simulink model "quad_1_ref_NN"  (R2018b)
settings: Solver=VariableStepAuto  StartTime=0.0  StopTime=20  RelTol=1e-3
undefined symbols (not defined in the file or in its folder): options
libraries: neural x348, simulink x3
(part 5 of 13)

== system quad_1_ref_NN/nn_1/Layer 3/Delays 1 ==
  "p{3}" : Inport  PortDimensions=30
      mask Display: e = 0.06;c1 = [120 230 180]/255;c2 = ([120 230 180]+0)/(256+128);c3 = ([120 230 180]+128)/(256+128);patch([0 1 1 0],[0 0 1 1],c1);patch([0 1 1 1-e 1-e 0+e],[0 0 1 1-e 0+e 0+e],c2);patch([0 0 1 1-e 0+e 0+e],[0 1 1 1-e 1-e 0+e],c3);plot([0 1 1 0 0],[0 0 1 1 0]);
  mux : Mux  Inputs=1
      mask Display: e = 0.06;c1 = [120 150 230]/255;c2 = ([120 150 230]+0)/383;c3 = ([120 150 230]+128)/383;patch([0 1 1 0],[0 0 1 1],c1);patch([0 1 1 1-e 1-e 0+e],[0 0 1 1-e 0+e 0+e],c2);patch([0 0 1 1-e 0+e 0+e],[0 1 1 1-e 1-e 0+e],c3);plot([0 1 1 0 0],[0 0 1 1 0]);disp('Mux')
  "pd{3,2}" : Outport
      mask Display: e = 0.06;c1 = [120 230 180]/255;c2 = ([120 230 180]+0)/(256+128);c3 = ([120 230 180]+128)/(256+128);patch([0 1 1 0],[0 0 1 1],c1);patch([0 1 1 1-e 1-e 0+e],[0 0 1 1-e 0+e 0+e],c2);patch([0 0 1 1-e 0+e 0+e],[0 1 1 1-e 1-e 0+e],c3);plot([0 1 1 0 0],[0 0 1 1 0]);
  wires:
  "p{3}"/1 -> mux/1
  mux/1 -> "pd{3,2}"/1

== system quad_1_ref_NN/nn_1/Layer 3/LW{3,2} ==
  "ad{3,2}" : Inport  PortDimensions=30
      mask Display: e = 0.06;c1 = [120 230 180]/255;c2 = ([120 230 180]+0)/(256+128);c3 = ([120 230 180]+128)/(256+128);patch([0 1 1 0],[0 0 1 1],c1);patch([0 1 1 1-e 1-e 0+e],[0 0 1 1-e 0+e 0+e],c2);patch([0 0 1 1-e 0+e 0+e],[0 1 1 1-e 1-e 0+e],c3);plot([0 1 1 0 0],[0 0 1 1 0]);
  "IW{3,2}(1,:)'" : Constant  Value=[0.276945469071661454218968856366700492799282073974609375;-0.30202511226643291575300054319086484611034393310546875;-0.20444458747253602126647820114158093929290771484375;-0.293398521295770098316069152133422903716564178466796875;-0.311767883755503738552050663201953284442424774169921875;0.2018687666357379117965109571741777472198009490966796875;-0.1423334383288296922653870524300145916640758514404296875;0.042721362346013591615445648130844347178936004638671875;-0.2329868918425182788833893710034317336976528167724609375;0.3249510619125837163068126756115816533565521240234375;-0.236296700940786752465072595441597513854503631591796875;0.0895607189297012162843003579837386496365070343017578125;0.12291057624967384465097808288192027248442173004150390625;-0.23707638583951962107931876744260080158710479736328125;-0.0601267258706521812161582829503458924591541290283203125;0.0826306713186458485775887083946145139634609222412109375;0.180972528352075279212129998995806090533733367919921875;-0.1529426971898099341107268855921574868261814117431640625;-0.2028170626333564430243683318622061051428318023681640625;0.1491957272053341110318314122196170501410961151123046875;0.170336272776724972910500355283147655427455902099609375;-0.28514001098319774474276755427126772701740264892578125;-0.1635604930433562642644318430029670707881450653076171875;0.360323245380352485955910424308967776596546173095703125;-0.349567524080722058510417582510854117572307586669921875;0.230681480735392574477060634308145381510257720947265625;0.2623154158955223191895811396534554660320281982421875;0.039798895545825989372712427893929998390376567840576171875;0.1587870984716829581007146998672396875917911529541015625;-0.26822414961531659827187468181364238262176513671875]
      mask Display: e = 0.06;c1 = [120 150 230]/255;c2 = ([120 150 230]+0)/383;c3 = ([120 150 230]+128)/383;patch([0 1 1 0],[0 0 1 1],c1);patch([0 1 1 1-e 1-e 0+e],[0 0 1 1-e 0+e 0+e],c2);patch([0 0 1 1-e 0+e 0+e],[0 1 1 1-e 1-e 0+e],c3);plot([0 1 1 0 0],[0 0 1 1 0]);disp('weights');
  "IW{3,2}(2,:)'" : Constant  Value=[-0.03253994981968925948034865314184571616351604461669921875;0.0550317097961975643105603239746415056288242340087890625;0.00642099379508191507592851365870956215076148509979248046875;0.03913085661204451781713942182250320911407470703125;-0.00475663585868581727245096857359385467134416103363037109375;-0.01086399947620869492481698870278705726377665996551513671875;0.0311382195567674602276753148544230498373508453369140625;-0.00372679100208476825339953819593574735336005687713623046875;-0.002270132986024297160054796762551632127724587917327880859375;0.020055220330963123565037875550842727534472942352294921875;0.0131234617942851128358228152137598954141139984130859375;0.0034257306991433904112820396647975940140895545482635498046875;-0.002660691719241682455521225136862994986586272716522216796875;0.0037828286499629027415936288747388971387408673763275146484375;-0.020157961923446821028704789569019339978694915771484375;-0.05222008698724234232457774851354770362377166748046875;-0.0196956397109985283100375141884796903468668460845947265625;0.021014223419305817774915823292758432216942310333251953125;-0.028243561683475686130417869890152360312640666961669921875;-0.0217372382094138498487279065329857985489070415496826171875;-0.0135213933507876242490208795743455993942916393280029296875;-0.00476408825410913443210159101681711035780608654022216796875;-0.00653767842271109345109181276711751706898212432861328125;-0.000516617713027289586491530570810937206260859966278076171875;0.024000774270628875972644067360306507907807826995849609375;0.01625825744361460156728327319797244854271411895751953125;-0.0030105080437037141059819500554795013158582150936126708984375;-0.0178769935667331854312056549360931967385113239288330078125;0.0523806529586079150373478796609560959041118621826171875;-0.0290655000588837496289240647229235037229955196380615234375]
      mask Display: e = 0.06;c1 = [120 150 230]/255;c2 = ([120 150 230]+0)/383;c3 = ([120 150 230]+128)/383;patch([0 1 1 0],[0 0 1 1],c1);patch([0 1 1 1-e 1-e 0+e],[0 0 1 1-e 0+e 0+e],c2);patch([0 0 1 1-e 0+e 0+e],[0 1 1 1-e 1-e 0+e],c3);plot([0 1 1 0 0],[0 0 1 1 0]);disp('weights');
  "IW{3,2}(3,:)'" : Constant  Value=[-0.009031921548045683534322591867748997174203395843505859375;0.05112964354185862980717303116762195713818073272705078125;0.022652209907742172634304012035499908961355686187744140625;0.04418223617098011868353779618701082654297351837158203125;-0.03234466873359742589144616431440226733684539794921875;0.0062948422769956470512742185974275344051420688629150390625;0.0075733059480824101161733352682858821935951709747314453125;-0.0031465398829118623909295582308232042123563587665557861328125;0.0257908390726858359476292292811194784007966518402099609375;0.01442129708941418224366071143549561384133994579315185546875;-0.003383104425635254097759485603091889061033725738525390625;0.01580392529714715055266793797272839583456516265869140625;-0.0310251890936021727795957048101627151481807231903076171875;-0.01179788359657658360080123571833610185422003269195556640625;-0.010215859514722404333131322573535726405680179595947265625;-0.05484074893927239069402190807522856630384922027587890625;-0.013821153985895277827022908923026989214122295379638671875;0.025982866454749765916520942710121744312345981597900390625;-0.021905026659969996372101519455100060440599918365478515625;-0.0526800415654134768228544771773158572614192962646484375;0.01189509994522582568554636139879221445880830287933349609375;0.01084111337574418000573306386513650068081915378570556640625;-0.00337372300491556829926675931119461893104016780853271484375;0.00449380387199421228727747035236461670137941837310791015625;0.0106078987897606606682909813343940186314284801483154296875;-0.00067881771438273175167665840490371920168399810791015625;-0.00932376731050502290110149061774791334755718708038330078125;-0.0245059899770730983681321646372452960349619388580322265625;0.019977292170611275767821979343352722935378551483154296875;-0.04273760279662632000086119887782842852175235748291015625]
      mask Display: e = 0.06;c1 = [120 150 230]/255;c2 = ([120 150 230]+0)/383;c3 = ([120 150 230]+128)/383;patch([0 1 1 0],[0 0 1 1],c1);patch([0 1 1 1-e 1-e 0+e],[0 0 1 1-e 0+e 0+e],c2);patch([0 0 1 1-e 0+e 0+e],[0 1 1 1-e 1-e 0+e],c3);plot([0 1 1 0 0],[0 0 1 1 0]);disp('weights');
  Mux : Mux  Inputs=3
      mask Display: e = 0.06;c1 = [120 150 230]/255;c2 = ([120 150 230]+0)/383;c3 = ([120 150 230]+128)/383;patch([0 1 1 0],[0 0 1 1],c1);patch([0 1 1 1-e 1-e 0+e],[0 0 1 1-e 0+e 0+e],c2);patch([0 0 1 1-e 0+e 0+e],[0 1 1 1-e 1-e 0+e],c3);plot([0 1 1 0 0],[0 0 1 1 0]);disp('Mux');
  dotprod1 : neural/Weight Functions/dotprod
  dotprod2 : neural/Weight Functions/dotprod
  dotprod3 : neural/Weight Functions/dotprod
  "lz{3,2}" : Outport
      mask Display: e = 0.06;c1 = [120 230 180]/255;c2 = ([120 230 180]+0)/(256+128);c3 = ([120 230 180]+128)/(256+128);patch([0 1 1 0],[0 0 1 1],c1);patch([0 1 1 1-e 1-e 0+e],[0 0 1 1-e 0+e 0+e],c2);patch([0 0 1 1-e 0+e 0+e],[0 1 1 1-e 1-e 0+e],c3);plot([0 1 1 0 0],[0 0 1 1 0]);
  wires:
  "IW{3,2}(1,:)'"/1 -> dotprod1/1
  "ad{3,2}"/1 -> dotprod1/2, dotprod2/2, dotprod3/2
  dotprod1/1 -> Mux/1
  "IW{3,2}(2,:)'"/1 -> dotprod2/1
  dotprod2/1 -> Mux/2
  "IW{3,2}(3,:)'"/1 -> dotprod3/1
  dotprod3/1 -> Mux/3
  Mux/1 -> "lz{3,2}"/1

== system quad_1_ref_NN/nn_1_const/Layer 1/Delays 1 ==
  "p{1}" : Inport  PortDimensions=12
      mask Display: e = 0.06;c1 = [120 230 180]/255;c2 = ([120 230 180]+0)/(256+128);c3 = ([120 230 180]+128)/(256+128);patch([0 1 1 0],[0 0 1 1],c1);patch([0 1 1 1-e 1-e 0+e],[0 0 1 1-e 0+e 0+e],c2);patch([0 0 1 1-e 0+e 0+e],[0 1 1 1-e 1-e 0+e],c3);plot([0 1 1 0 0],[0 0 1 1 0]);
  mux : Mux  Inputs=1
      mask Display: e = 0.06;c1 = [120 150 230]/255;c2 = ([120 150 230]+0)/383;c3 = ([120 150 230]+128)/383;patch([0 1 1 0],[0 0 1 1],c1);patch([0 1 1 1-e 1-e 0+e],[0 0 1 1-e 0+e 0+e],c2);patch([0 0 1 1-e 0+e 0+e],[0 1 1 1-e 1-e 0+e],c3);plot([0 1 1 0 0],[0 0 1 1 0]);disp('Mux')
  "pd{1,1}" : Outport
      mask Display: e = 0.06;c1 = [120 230 180]/255;c2 = ([120 230 180]+0)/(256+128);c3 = ([120 230 180]+128)/(256+128);patch([0 1 1 0],[0 0 1 1],c1);patch([0 1 1 1-e 1-e 0+e],[0 0 1 1-e 0+e 0+e],c2);patch([0 0 1 1-e 0+e 0+e],[0 1 1 1-e 1-e 0+e],c3);plot([0 1 1 0 0],[0 0 1 1 0]);
  wires:
  "p{1}"/1 -> mux/1
  mux/1 -> "pd{1,1}"/1

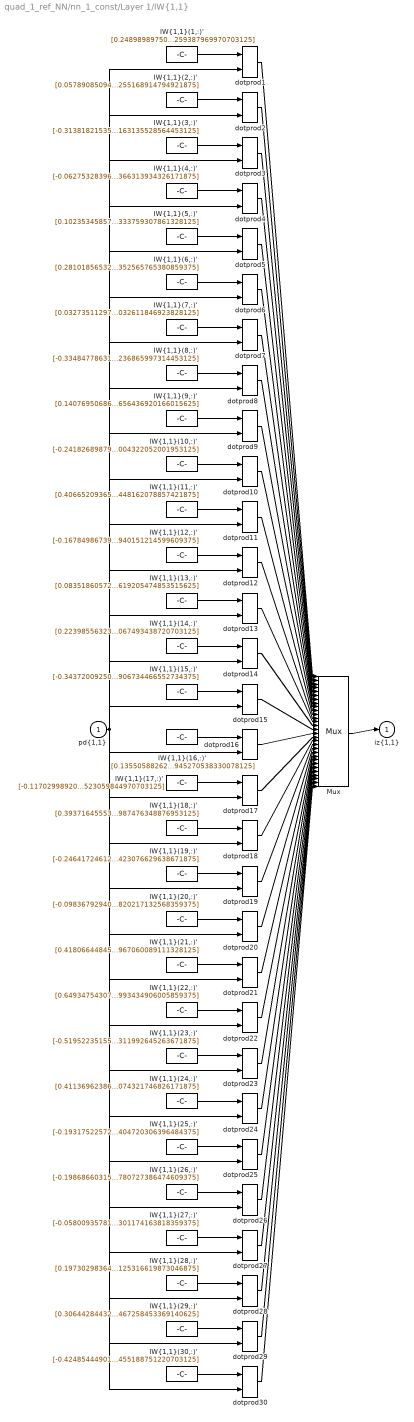
== system quad_1_ref_NN/nn_1_const/Layer 1/IW{1,1} ==
  "pd{1,1}" : Inport  PortDimensions=12
      mask Display: e = 0.06;c1 = [120 230 180]/255;c2 = ([120 230 180]+0)/(256+128);c3 = ([120 230 180]+128)/(256+128);patch([0 1 1 0],[0 0 1 1],c1);patch([0 1 1 1-e 1-e 0+e],[0 0 1 1-e 0+e 0+e],c2);patch([0 0 1 1-e 0+e 0+e],[0 1 1 1-e 1-e 0+e],c3);plot([0 1 1 0 0],[0 0 1 1 0]);
  "IW{1,1}(1,:)'" : Constant  Value=[0.2489898975063435937471467696013860404491424560546875;-0.112298286921174328423234101137495599687099456787109375;-0.041923837097128206774510061904948088340461254119873046875;-0.046673404176335420157073485825094394385814666748046875;0.432665213666946379955646762027754448354244232177734375;-0.0097132578185999095266023317662984482012689113616943359375;0.32656184582790304116173274451284669339656829833984375;0.11158683144684687638115150321027613244950771331787109375;-0.00174609248808417038927032205464229264180175960063934326171875;0.424027280725470578914837460615672171115875244140625;0.458406862610547083392020795145072042942047119140625;-0.0370983845065871176149840948710334487259387969970703125]
      mask Display: e = 0.06;c1 = [120 150 230]/255;c2 = ([120 150 230]+0)/383;c3 = ([120 150 230]+128)/383;patch([0 1 1 0],[0 0 1 1],c1);patch([0 1 1 1-e 1-e 0+e],[0 0 1 1-e 0+e 0+e],c2);patch([0 0 1 1-e 0+e 0+e],[0 1 1 1-e 1-e 0+e],c3);plot([0 1 1 0 0],[0 0 1 1 0]);disp('Weights');
  "IW{1,1}(10,:)'" : Constant  Value=[-0.241826898792885547351261266157962381839752197265625;0.3919254723671212747859726732713170349597930908203125;-0.0213357064703371020197852914179748040623962879180908203125;-0.09792977901171183441331180574707104824483394622802734375;0.047839481153725486872740901844736072234809398651123046875;0.116526714482541871031884284093393944203853607177734375;-0.0918185950644110626672755870458786375820636749267578125;-0.197897683283946912435879994518472813069820404052734375;-0.0712123900064262349562937970404163934290409088134765625;-0.34083989126823810433819517129450105130672454833984375;-0.56405002922402591725159481939044781029224395751953125;0.031834197805936444158891873712491360493004322052001953125]
      mask Display: e = 0.06;c1 = [120 150 230]/255;c2 = ([120 150 230]+0)/383;c3 = ([120 150 230]+128)/383;patch([0 1 1 0],[0 0 1 1],c1);patch([0 1 1 1-e 1-e 0+e],[0 0 1 1-e 0+e 0+e],c2);patch([0 0 1 1-e 0+e 0+e],[0 1 1 1-e 1-e 0+e],c3);plot([0 1 1 0 0],[0 0 1 1 0]);disp('Weights');
  "IW{1,1}(11,:)'" : Constant  Value=[0.406652093651284685105196103904745541512966156005859375;-0.276759606675215596993666622438468039035797119140625;-0.1913370529300668920757999558190931566059589385986328125;0.311012617222419240903263926156796514987945556640625;-0.18175282140661253027502652912517078220844268798828125;-0.05621199948579279348503945357151678763329982757568359375;0.207761145657090418037427070885314606130123138427734375;0.29617604491022142543243944601272232830524444580078125;-0.2494736920950384462258853091043420135974884033203125;-0.398387101331069859444511394030996598303318023681640625;0.37593373815508146496000563274719752371311187744140625;0.0935813620128422563038128600965137593448162078857421875]
      mask Display: e = 0.06;c1 = [120 150 230]/255;c2 = ([120 150 230]+0)/383;c3 = ([120 150 230]+128)/383;patch([0 1 1 0],[0 0 1 1],c1);patch([0 1 1 1-e 1-e 0+e],[0 0 1 1-e 0+e 0+e],c2);patch([0 0 1 1-e 0+e 0+e],[0 1 1 1-e 1-e 0+e],c3);plot([0 1 1 0 0],[0 0 1 1 0]);disp('Weights');
  "IW{1,1}(12,:)'" : Constant  Value=[-0.1678498673909872007659060955120366998016834259033203125;0.30057791076311601852211197183351032435894012451171875;-0.2068623881193169811165688543042051605880260467529296875;0.03127024359038514667030739246911252848803997039794921875;-0.275997240372790997309238036905298940837383270263671875;0.366594694572909662877435721384244970977306365966796875;0.4295578731804960970208639992051757872104644775390625;0.327463701071572355072447635393473319709300994873046875;-0.193276403110250794004087993016582913696765899658203125;-0.345485768180975372221297448049881495535373687744140625;-0.1335022226039513648654377675484283827245235443115234375;0.1217009352881620320996347572872764430940151214599609375]
      mask Display: e = 0.06;c1 = [120 150 230]/255;c2 = ([120 150 230]+0)/383;c3 = ([120 150 230]+128)/383;patch([0 1 1 0],[0 0 1 1],c1);patch([0 1 1 1-e 1-e 0+e],[0 0 1 1-e 0+e 0+e],c2);patch([0 0 1 1-e 0+e 0+e],[0 1 1 1-e 1-e 0+e],c3);plot([0 1 1 0 0],[0 0 1 1 0]);disp('Weights');
  "IW{1,1}(13,:)'" : Constant  Value=[0.08351860572411019811855936723077320493757724761962890625;-0.413325214603568025228952365068835206329822540283203125;-0.302060946120565165795568418616312555968761444091796875;-0.116192348966924707820425055615487508475780487060546875;-0.149872004616036225144171112333424389362335205078125;0.3732993546496150560898286130395717918872833251953125;-0.44533869376238433002157535156584344804286956787109375;0.0395748086544917831997025814416701905429363250732421875;0.1197405812416630632721847860011621378362178802490234375;-0.41575965708720274971454955448280088603496551513671875;-0.2246661150830329967131859802975668571889400482177734375;-0.0216388332703475738671983208405436016619205474853515625]
      mask Display: e = 0.06;c1 = [120 150 230]/255;c2 = ([120 150 230]+0)/383;c3 = ([120 150 230]+128)/383;patch([0 1 1 0],[0 0 1 1],c1);patch([0 1 1 1-e 1-e 0+e],[0 0 1 1-e 0+e 0+e],c2);patch([0 0 1 1-e 0+e 0+e],[0 1 1 1-e 1-e 0+e],c3);plot([0 1 1 0 0],[0 0 1 1 0]);disp('Weights');
  "IW{1,1}(14,:)'" : Constant  Value=[0.223985563232536766253844007223960943520069122314453125;-0.04945192503423155583330839135669521056115627288818359375;-0.1962965394305775934657987136233714409172534942626953125;0.0295316519582797358534076437308613094501197338104248046875;0.07949822490435536070929600782619672827422618865966796875;-0.51816763343045213474624688387848436832427978515625;0.10949461368816186535024570503082941286265850067138671875;-0.01143505829141123163184001754189011990092694759368896484375;0.582963912201748701846781841595657169818878173828125;0.0268494871259278948538717912697393330745398998260498046875;0.0069103283755132215160355002581127337180078029632568359375;-0.4759050293050759439239527637255378067493438720703125]
      mask Display: e = 0.06;c1 = [120 150 230]/255;c2 = ([120 150 230]+0)/383;c3 = ([120 150 230]+128)/383;patch([0 1 1 0],[0 0 1 1],c1);patch([0 1 1 1-e 1-e 0+e],[0 0 1 1-e 0+e 0+e],c2);patch([0 0 1 1-e 0+e 0+e],[0 1 1 1-e 1-e 0+e],c3);plot([0 1 1 0 0],[0 0 1 1 0]);disp('Weights');
  "IW{1,1}(15,:)'" : Constant  Value=[-0.34372009250453372519729100531549192965030670166015625;-0.3295648638163488630681285940227098762989044189453125;-0.26076996190842560707778829964809119701385498046875;-0.0354217042376119561897240828329813666641712188720703125;-0.32720899914815737563600350767956115305423736572265625;-0.2344401070546141274686391398063278757035732269287109375;-0.340184475584872914044609615302761085331439971923828125;-0.27627829555073779577156756204203702509403228759765625;0.1048058417402470687829207918184692971408367156982421875;-0.15736575485780124328272222555824555456638336181640625;0.334995769922207198288077734105172567069530487060546875;0.1470607822368401595980458296253345906734466552734375]
      mask Display: e = 0.06;c1 = [120 150 230]/255;c2 = ([120 150 230]+0)/383;c3 = ([120 150 230]+128)/383;patch([0 1 1 0],[0 0 1 1],c1);patch([0 1 1 1-e 1-e 0+e],[0 0 1 1-e 0+e 0+e],c2);patch([0 0 1 1-e 0+e 0+e],[0 1 1 1-e 1-e 0+e],c3);plot([0 1 1 0 0],[0 0 1 1 0]);disp('Weights');
  "IW{1,1}(16,:)'" : Constant  Value=[0.1355058826287278972433369972350192256271839141845703125;-0.327508281343989182676779137182165868580341339111328125;-0.162426252210169097534020465900539420545101165771484375;-0.379662675760057855001150528551079332828521728515625;-0.02615657306319595087895635288077755831182003021240234375;0.2034431436294713291257352238972089253365993499755859375;0.0037668162158365713597374391241601188085041940212249755859375;-0.386785824856337001609318804185022599995136260986328125;-0.08908442379376861619544314407903584651648998260498046875;0.419719320235534099072793878804077394306659698486328125;-0.394700658331529175004703802187577821314334869384765625;0.06888911276263716410017678981603239662945270538330078125]
      mask Display: e = 0.06;c1 = [120 150 230]/255;c2 = ([120 150 230]+0)/383;c3 = ([120 150 230]+128)/383;patch([0 1 1 0],[0 0 1 1],c1);patch([0 1 1 1-e 1-e 0+e],[0 0 1 1-e 0+e 0+e],c2);patch([0 0 1 1-e 0+e 0+e],[0 1 1 1-e 1-e 0+e],c3);plot([0 1 1 0 0],[0 0 1 1 0]);disp('Weights');
  "IW{1,1}(17,:)'" : Constant  Value=[-0.11702998920231670598735007615687209181487560272216796875;0.165125718981726177236879493648302741348743438720703125;0.377746972276425563297408416474354453384876251220703125;0.285586546046543376942139502716599963605403900146484375;-0.1983913236010440284129430210668942891061305999755859375;0.11105872652019599389205950501491315662860870361328125;-0.37393787900743202801123743483913131058216094970703125;0.26784833233075400205080995874595828354358673095703125;0.1591137251703405031122429136303253471851348876953125;0.36483860541726864656908446704619564116001129150390625;-0.452102401579462076508519885464920662343502044677734375;0.101835814179770889342790951559436507523059844970703125]
      mask Display: e = 0.06;c1 = [120 150 230]/255;c2 = ([120 150 230]+0)/383;c3 = ([120 150 230]+128)/383;patch([0 1 1 0],[0 0 1 1],c1);patch([0 1 1 1-e 1-e 0+e],[0 0 1 1-e 0+e 0+e],c2);patch([0 0 1 1-e 0+e 0+e],[0 1 1 1-e 1-e 0+e],c3);plot([0 1 1 0 0],[0 0 1 1 0]);disp('Weights');
  "IW{1,1}(18,:)'" : Constant  Value=[0.3937164555378875885338629814214073121547698974609375;0.1434135429879584699985883844419731758534908294677734375;0.028038542485958127536971318249925388954579830169677734375;-0.036970753832619100698320124820384080521762371063232421875;-0.32516652988799155110655192402191460132598876953125;0.1050337733726433853131965179272810928523540496826171875;0.61974287674472339215725469330209307372570037841796875;-0.23204538935426644030712850508280098438262939453125;-0.01487323798730660028011296702743493369780480861663818359375;0.419962473587843165834243563949712552130222320556640625;-0.03262480095089526077600794451427645981311798095703125;0.01765178315032940592477217478517559356987476348876953125]
      mask Display: e = 0.06;c1 = [120 150 230]/255;c2 = ([120 150 230]+0)/383;c3 = ([120 150 230]+128)/383;patch([0 1 1 0],[0 0 1 1],c1);patch([0 1 1 1-e 1-e 0+e],[0 0 1 1-e 0+e 0+e],c2);patch([0 0 1 1-e 0+e 0+e],[0 1 1 1-e 1-e 0+e],c3);plot([0 1 1 0 0],[0 0 1 1 0]);disp('Weights');
  "IW{1,1}(19,:)'" : Constant  Value=[-0.2464172461222495502664031619133311323821544647216796875;0.04603839551253331718871919520097435452044010162353515625;-0.406619982447500138977858341604587621986865997314453125;-0.08767248588044539159280787998795858584344387054443359375;0.427889669285226370565311526661389507353305816650390625;0.233577623244786314327114951083785854279994964599609375;-0.00594801069686133436487107672974161687307059764862060546875;0.2428804997477155003249293940825737081468105316162109375;0.18109123859714859605674064368940889835357666015625;-0.241228406468116107763677291586645878851413726806640625;-0.327213535918858433593214840584550984203815460205078125;-0.25539225792708719620094370839069597423076629638671875]
      mask Display: e = 0.06;c1 = [120 150 230]/255;c2 = ([120 150 230]+0)/383;c3 = ([120 150 230]+128)/383;patch([0 1 1 0],[0 0 1 1],c1);patch([0 1 1 1-e 1-e 0+e],[0 0 1 1-e 0+e 0+e],c2);patch([0 0 1 1-e 0+e 0+e],[0 1 1 1-e 1-e 0+e],c3);plot([0 1 1 0 0],[0 0 1 1 0]);disp('Weights');
  "IW{1,1}(2,:)'" : Constant  Value=[0.05789085094579828061345239120782935060560703277587890625;-0.035820270835119571994908937995205633342266082763671875;-0.1086830227150221428455978411875548772513866424560546875;0.1759710014715628323411777955698198638856410980224609375;-0.127833816484399509505465175607241690158843994140625;-0.23864940102912601815887683187611401081085205078125;-0.5915594204225589347601044210023246705532073974609375;-0.3954211523158603913685738007188774645328521728515625;-0.0611826492362775586908441027844673953950405120849609375;-0.0764974144790842858210311305811046622693538665771484375;0.2051401418239207352645081527953152544796466827392578125;0.35786936592520823818830422169412486255168914794921875]
      mask Display: e = 0.06;c1 = [120 150 230]/255;c2 = ([120 150 230]+0)/383;c3 = ([120 150 230]+128)/383;patch([0 1 1 0],[0 0 1 1],c1);patch([0 1 1 1-e 1-e 0+e],[0 0 1 1-e 0+e 0+e],c2);patch([0 0 1 1-e 0+e 0+e],[0 1 1 1-e 1-e 0+e],c3);plot([0 1 1 0 0],[0 0 1 1 0]);disp('Weights');
  "IW{1,1}(20,:)'" : Constant  Value=[-0.098367929400794140715191815615980885922908782958984375;0.342954572931524481749221422433038242161273956298828125;0.388210390152917472761373574030585587024688720703125;-0.289753967523580679976902274574968032538890838623046875;0.11030854882083428181172024551415233872830867767333984375;0.35627456599792084457334340186207555234432220458984375;-0.37551785170355811427356229614815674722194671630859375;-0.1010387180394585471265855858291615732014179229736328125;0.0157785920497450458943600182237787521444261074066162109375;0.0761227164492360997005704348339349962770938873291015625;0.040635956122396142686792330778189352713525295257568359375;0.39966097433820946260851769693545065820217132568359375]
      mask Display: e = 0.06;c1 = [120 150 230]/255;c2 = ([120 150 230]+0)/383;c3 = ([120 150 230]+128)/383;patch([0 1 1 0],[0 0 1 1],c1);patch([0 1 1 1-e 1-e 0+e],[0 0 1 1-e 0+e 0+e],c2);patch([0 0 1 1-e 0+e 0+e],[0 1 1 1-e 1-e 0+e],c3);plot([0 1 1 0 0],[0 0 1 1 0]);disp('Weights');
  "IW{1,1}(21,:)'" : Constant  Value=[0.418066448451700656274709899662411771714687347412109375;0.19848114693118723561582328329677693545818328857421875;0.322774437159183358314606948624714277684688568115234375;-0.47652777901823462070041159677202813327312469482421875;0.2428207792046696844590059072288568131625652313232421875;-0.0804763626894953454371517409526859410107135772705078125;0.293151927406080037297186891009914688766002655029296875;0.291116712625121232260738679542555473744869232177734375;-0.254803823380726990333045023362501524388790130615234375;0.2039600205682643163651590612062136642634868621826171875;0.2484758258771164463052372184392879717051982879638671875;-0.277128631572702233132332594323088414967060089111328125]
      mask Display: e = 0.06;c1 = [120 150 230]/255;c2 = ([120 150 230]+0)/383;c3 = ([120 150 230]+128)/383;patch([0 1 1 0],[0 0 1 1],c1);patch([0 1 1 1-e 1-e 0+e],[0 0 1 1-e 0+e 0+e],c2);patch([0 0 1 1-e 0+e 0+e],[0 1 1 1-e 1-e 0+e],c3);plot([0 1 1 0 0],[0 0 1 1 0]);disp('Weights');
  "IW{1,1}(22,:)'" : Constant  Value=[0.64934754307484376933956582433893345296382904052734375;-0.062206259378859769804126500503116403706371784210205078125;0.266999388289536898621889804417151026427745819091796875;0.0807890814383341593352128029437153600156307220458984375;-0.0204002869299817757298143305888515897095203399658203125;0.049077715375807129394303274239064194262027740478515625;-0.288515373202615499348411276514525525271892547607421875;0.216290515567391594675683563764323480427265167236328125;-0.410134786815746277266470087852212600409984588623046875;-0.291970449183066527165664183485205285251140594482421875;0.273417705144658962357340215021395124495029449462890625;-0.092430862968949367708404452059767208993434906005859375]
      mask Display: e = 0.06;c1 = [120 150 230]/255;c2 = ([120 150 230]+0)/383;c3 = ([120 150 230]+128)/383;patch([0 1 1 0],[0 0 1 1],c1);patch([0 1 1 1-e 1-e 0+e],[0 0 1 1-e 0+e 0+e],c2);patch([0 0 1 1-e 0+e 0+e],[0 1 1 1-e 1-e 0+e],c3);plot([0 1 1 0 0],[0 0 1 1 0]);disp('Weights');
  "IW{1,1}(23,:)'" : Constant  Value=[-0.5195223515554598936461161429178901016712188720703125;0.00798812362191856674409340399733991944231092929840087890625;0.321155453014911607123593739743228070437908172607421875;0.1470597592653031526754858759886701591312885284423828125;0.1567351397212360664124020104281953535974025726318359375;0.31655013993840708241833681313437409698963165283203125;0.461043494324328728684037059792899526655673980712890625;-0.02602690496373905038041129955672658979892730712890625;0.252863699844429579144389208522625267505645751953125;0.11872854218900928680024975392370834015309810638427734375;0.225971343919305789338380918707116506993770599365234375;0.157608321730608735844469947551260702311992645263671875]
      mask Display: e = 0.06;c1 = [120 150 230]/255;c2 = ([120 150 230]+0)/383;c3 = ([120 150 230]+128)/383;patch([0 1 1 0],[0 0 1 1],c1);patch([0 1 1 1-e 1-e 0+e],[0 0 1 1-e 0+e 0+e],c2);patch([0 0 1 1-e 0+e 0+e],[0 1 1 1-e 1-e 0+e],c3);plot([0 1 1 0 0],[0 0 1 1 0]);disp('Weights');
  "IW{1,1}(24,:)'" : Constant  Value=[0.41136962386269815272754613033612258732318878173828125;-0.00986684331039336219582036591191354091279208660125732421875;-0.1692049635383326700033279621493420563638210296630859375;0.2853137061805390839452911677653901278972625732421875;-0.25557693030708861225974715125630609691143035888671875;0.38587525561457980405322132355649955570697784423828125;-0.161212833221031470731787749173236079514026641845703125;0.004202460895385063711915396567064817645587027072906494140625;0.388387531978571620694395960526890121400356292724609375;0.271117782220159142525517381727695465087890625;-0.32612873356319027617900019322405569255352020263671875;-0.243028019876800172038855407663504593074321746826171875]
      mask Display: e = 0.06;c1 = [120 150 230]/255;c2 = ([120 150 230]+0)/383;c3 = ([120 150 230]+128)/383;patch([0 1 1 0],[0 0 1 1],c1);patch([0 1 1 1-e 1-e 0+e],[0 0 1 1-e 0+e 0+e],c2);patch([0 0 1 1-e 0+e 0+e],[0 1 1 1-e 1-e 0+e],c3);plot([0 1 1 0 0],[0 0 1 1 0]);disp('Weights');
  "IW{1,1}(25,:)'" : Constant  Value=[-0.1931752257265579031386693031890899874269962310791015625;0.3449778258577869127776693858322687447071075439453125;0.0974488225591378098844330679639824666082859039306640625;-0.033452684219077065408409765723263262771070003509521484375;0.325049336493253182567286785342730581760406494140625;-0.346622946305623014229269074348849244415760040283203125;0.36423747104963510867747800148208625614643096923828125;0.219000556930524170606844336361973546445369720458984375;0.374508049470750503662230812551570124924182891845703125;0.2334799563788132470421032849117182195186614990234375;-0.01693188442818571726178333847201429307460784912109375;0.0369551622368794185913287719813524745404720306396484375]
      mask Display: e = 0.06;c1 = [120 150 230]/255;c2 = ([120 150 230]+0)/383;c3 = ([120 150 230]+128)/383;patch([0 1 1 0],[0 0 1 1],c1);patch([0 1 1 1-e 1-e 0+e],[0 0 1 1-e 0+e 0+e],c2);patch([0 0 1 1-e 0+e 0+e],[0 1 1 1-e 1-e 0+e],c3);plot([0 1 1 0 0],[0 0 1 1 0]);disp('Weights');
  "IW{1,1}(26,:)'" : Constant  Value=[-0.198686603157890051551959231801447458565235137939453125;0.342046774450926294175445718792616389691829681396484375;0.09653772198672432025556844337188522331416606903076171875;-0.3587007705305200744305693660862743854522705078125;-0.37833647195315156519512811428285203874111175537109375;0.145511619763073252187268735724501311779022216796875;-0.206050731708805889841329417322413064539432525634765625;-0.278386570100078500900053768418729305267333984375;-0.063551947240046757769960095174610614776611328125;0.430597821957975634976634182748966850340366363525390625;0.2409602060956436975214245421739178709685802459716796875;0.1277127284068340917766448683323687873780727386474609375]
      mask Display: e = 0.06;c1 = [120 150 230]/255;c2 = ([120 150 230]+0)/383;c3 = ([120 150 230]+128)/383;patch([0 1 1 0],[0 0 1 1],c1);patch([0 1 1 1-e 1-e 0+e],[0 0 1 1-e 0+e 0+e],c2);patch([0 0 1 1-e 0+e 0+e],[0 1 1 1-e 1-e 0+e],c3);plot([0 1 1 0 0],[0 0 1 1 0]);disp('Weights');
  "IW{1,1}(27,:)'" : Constant  Value=[-0.0580093578197561077214317037942237220704555511474609375;-0.386409681317652797805095588046242482960224151611328125;0.07981918628557473083251494472278864122927188873291015625;-0.31193748389987197011663511148071847856044769287109375;-0.2365185946105781977788495851200423203408718109130859375;0.4156781218510914310826365181128494441509246826171875;0.3428637849538773707536165602505207061767578125;-0.183299188191856199381390979397110641002655029296875;0.022086677472191403037715673463026178069412708282470703125;0.152336218501208431330695702854427509009838104248046875;-0.1456432016485578184727955886046402156352996826171875;0.356298422203449260958763034068397246301174163818359375]
      mask Display: e = 0.06;c1 = [120 150 230]/255;c2 = ([120 150 230]+0)/383;c3 = ([120 150 230]+128)/383;patch([0 1 1 0],[0 0 1 1],c1);patch([0 1 1 1-e 1-e 0+e],[0 0 1 1-e 0+e 0+e],c2);patch([0 0 1 1-e 0+e 0+e],[0 1 1 1-e 1-e 0+e],c3);plot([0 1 1 0 0],[0 0 1 1 0]);disp('Weights');
  "IW{1,1}(28,:)'" : Constant  Value=[0.1973029836404917858327934254702995531260967254638671875;0.0241500974368777550360665173911911551840603351593017578125;0.33809384578087087191988757695071399211883544921875;-0.213188326538220340733431612534332089126110076904296875;-0.301487765495815740468543708630022592842578887939453125;0.2017161404228234033997324559095432050526142120361328125;-0.364772400590195278180516424981760792434215545654296875;0.150952966704133328956771720186225138604640960693359375;-0.164927290226866307687458856889861635863780975341796875;0.43839633877965444863633592831320129334926605224609375;0.3644457298115548748995706773712299764156341552734375;-0.144852305373128042997876718800398521125316619873046875]
      mask Display: e = 0.06;c1 = [120 150 230]/255;c2 = ([120 150 230]+0)/383;c3 = ([120 150 230]+128)/383;patch([0 1 1 0],[0 0 1 1],c1);patch([0 1 1 1-e 1-e 0+e],[0 0 1 1-e 0+e 0+e],c2);patch([0 0 1 1-e 0+e 0+e],[0 1 1 1-e 1-e 0+e],c3);plot([0 1 1 0 0],[0 0 1 1 0]);disp('Weights');
  "IW{1,1}(29,:)'" : Constant  Value=[0.3064428443290843073754103897954337298870086669921875;0.1770597129549205950294066269634640775620937347412109375;-0.1469234198009608804991188435451476834714412689208984375;-0.27353269131383850520933265215717256069183349609375;0.0860404119337548622947764442869811318814754486083984375;-0.1463961528910358300681338050708291120827198028564453125;0.30788993004248832452418582761310972273349761962890625;-0.0511760982543132403321806123130954802036285400390625;0.0023318336522221388799891439447264929185621440410614013671875;-0.393518894563981203038594003373873420059680938720703125;-0.33741482017431401185802997133578173816204071044921875;0.359941389454050908458526691902079619467258453369140625]
      mask Display: e = 0.06;c1 = [120 150 230]/255;c2 = ([120 150 230]+0)/383;c3 = ([120 150 230]+128)/383;patch([0 1 1 0],[0 0 1 1],c1);patch([0 1 1 1-e 1-e 0+e],[0 0 1 1-e 0+e 0+e],c2);patch([0 0 1 1-e 0+e 0+e],[0 1 1 1-e 1-e 0+e],c3);plot([0 1 1 0 0],[0 0 1 1 0]);disp('Weights');
  "IW{1,1}(3,:)'" : Constant  Value=[-0.313818215353153184832279976035351864993572235107421875;0.029302649804127840760248346896332805044949054718017578125;0.15139671749946648215967570649809204041957855224609375;0.31085797834116402071913398685865104198455810546875;-0.43575083038882500563460098419454880058765411376953125;-0.3650054041928132431138465108233503997325897216796875;0.3879103620234596316862507592304609715938568115234375;-0.09982323619706369444148919001236208714544773101806640625;-0.0616286853050250493790684913619770668447017669677734375;0.03438861475803829670372380178378080017864704132080078125;-0.260832451652394270436019496628432534635066986083984375;0.0287224860061644944597691875287637230940163135528564453125]
      mask Display: e = 0.06;c1 = [120 150 230]/255;c2 = ([120 150 230]+0)/383;c3 = ([120 150 230]+128)/383;patch([0 1 1 0],[0 0 1 1],c1);patch([0 1 1 1-e 1-e 0+e],[0 0 1 1-e 0+e 0+e],c2);patch([0 0 1 1-e 0+e 0+e],[0 1 1 1-e 1-e 0+e],c3);plot([0 1 1 0 0],[0 0 1 1 0]);disp('Weights');
  "IW{1,1}(30,:)'" : Constant  Value=[-0.424854449015584112459009702433831989765167236328125;0.0067476005626217507027408970543547184206545352935791015625;0.3566408013223949513559318802435882389545440673828125;-0.326097950089787314009726060248794965445995330810546875;0.0809187204142436389275871988502331078052520751953125;0.35211914638322350246113501270883716642856597900390625;0.08420216401525547345041644575758255086839199066162109375;0.259244970462429280555483046555309556424617767333984375;-0.07338856981348958197219900512209278531372547149658203125;-0.31598032571246381650098555837757885456085205078125;0.31674711737494565255701672867871820926666259765625;0.0767244040276849059711850031817448325455188751220703125]
      mask Display: e = 0.06;c1 = [120 150 230]/255;c2 = ([120 150 230]+0)/383;c3 = ([120 150 230]+128)/383;patch([0 1 1 0],[0 0 1 1],c1);patch([0 1 1 1-e 1-e 0+e],[0 0 1 1-e 0+e 0+e],c2);patch([0 0 1 1-e 0+e 0+e],[0 1 1 1-e 1-e 0+e],c3);plot([0 1 1 0 0],[0 0 1 1 0]);disp('Weights');
  "IW{1,1}(4,:)'" : Constant  Value=[-0.0627532839624274918488566754604107700288295745849609375;0.4381621869335357022379184854798950254917144775390625;-0.077674906720971825802024568474735133349895477294921875;-0.20092737899488233299649664331809617578983306884765625;-0.329820365544929716694610988270142115652561187744140625;-0.12097622778736590032355735502278548665344715118408203125;-0.324835610884430414646573126447037793695926666259765625;0.17151183198656105854951192668522708117961883544921875;0.421960374163837970140633615301339887082576751708984375;-0.010243785313842936057771026980844908393919467926025390625;-0.0538114595021002284358502265604329295456409454345703125;0.34338332921234282490985378899495117366313934326171875]
      mask Display: e = 0.06;c1 = [120 150 230]/255;c2 = ([120 150 230]+0)/383;c3 = ([120 150 230]+128)/383;patch([0 1 1 0],[0 0 1 1],c1);patch([0 1 1 1-e 1-e 0+e],[0 0 1 1-e 0+e 0+e],c2);patch([0 0 1 1-e 0+e 0+e],[0 1 1 1-e 1-e 0+e],c3);plot([0 1 1 0 0],[0 0 1 1 0]);disp('Weights');
  "IW{1,1}(5,:)'" : Constant  Value=[0.1023534585701468546670156456457334570586681365966796875;-0.07203234098429291132337226599702262319624423980712890625;-0.264496400973797063382875194292864762246608734130859375;-0.447778834786195567563282793344114907085895538330078125;0.296580698126901187716697450014180503785610198974609375;-0.052646173338619504933344472874523489736020565032958984375;-0.259928010136457221523897942461189813911914825439453125;0.1302485987928166111249339564892579801380634307861328125;0.42710770370757844549558512881048955023288726806640625;0.02600930588150966726868063005895237438380718231201171875;-0.31493054111418106177922027200111187994480133056640625;-0.391904916462935404286582752320100553333759307861328125]
      mask Display: e = 0.06;c1 = [120 150 230]/255;c2 = ([120 150 230]+0)/383;c3 = ([120 150 230]+128)/383;patch([0 1 1 0],[0 0 1 1],c1);patch([0 1 1 1-e 1-e 0+e],[0 0 1 1-e 0+e 0+e],c2);patch([0 0 1 1-e 0+e 0+e],[0 1 1 1-e 1-e 0+e],c3);plot([0 1 1 0 0],[0 0 1 1 0]);disp('Weights');
  "IW{1,1}(6,:)'" : Constant  Value=[0.281018565325792446518704537083976902067661285400390625;0.22085522181168337763068620915873907506465911865234375;-0.1088500840754953180589126304766978137195110321044921875;-0.401339368623628900412114717255462892353534698486328125;0.26165922606231439839774566280539147555828094482421875;0.37578239746938446597113170355441980063915252685546875;-0.1425778078164375017866660755316843278706073760986328125;-0.028749934162471020571150148725791950710117816925048828125;-0.3740911003867040118819886629353277385234832763671875;-0.2346596477626363974611223284227889962494373321533203125;-0.34925379158177849436839323971071280539035797119140625;0.0806041574515269088063718072589836083352565765380859375]
      mask Display: e = 0.06;c1 = [120 150 230]/255;c2 = ([120 150 230]+0)/383;c3 = ([120 150 230]+128)/383;patch([0 1 1 0],[0 0 1 1],c1);patch([0 1 1 1-e 1-e 0+e],[0 0 1 1-e 0+e 0+e],c2);patch([0 0 1 1-e 0+e 0+e],[0 1 1 1-e 1-e 0+e],c3);plot([0 1 1 0 0],[0 0 1 1 0]);disp('Weights');
  "IW{1,1}(7,:)'" : Constant  Value=[0.032735112973678093251095333471312187612056732177734375;0.1633969542453883594390617872704751789569854736328125;0.3768755565440742305582944027264602482318878173828125;0.38481823547160931564548036476480774581432342529296875;-0.381971492925512745575389317309600301086902618408203125;0.07292115369071754116259143074785242788493633270263671875;0.37059347638131467927991025135270319879055023193359375;0.01770759446695902017410162443411536514759063720703125;0.135708258015824423381445740233175456523895263671875;0.1261946717109042881421743231840082444250583648681640625;-0.272802855991440995619967679886030964553356170654296875;0.24378833019334067433447899020393379032611846923828125]
      mask Display: e = 0.06;c1 = [120 150 230]/255;c2 = ([120 150 230]+0)/383;c3 = ([120 150 230]+128)/383;patch([0 1 1 0],[0 0 1 1],c1);patch([0 1 1 1-e 1-e 0+e],[0 0 1 1-e 0+e 0+e],c2);patch([0 0 1 1-e 0+e 0+e],[0 1 1 1-e 1-e 0+e],c3);plot([0 1 1 0 0],[0 0 1 1 0]);disp('Weights');
  "IW{1,1}(8,:)'" : Constant  Value=[-0.334847786318940465744020684724091552197933197021484375;-0.1957745987340176185842466338726808317005634307861328125;-0.09306069651897037886545405172000755555927753448486328125;0.057299836625843252047030063067722949199378490447998046875;-0.386536767099979028383671675328514538705348968505859375;-0.399168114120369177388880643775337375700473785400390625;0.2159646130252184936804127346476889215409755706787109375;0.04779640482843501569920618976539117284119129180908203125;0.329658145618675180177348238430568017065525054931640625;-0.2733967558765402205978034544386900961399078369140625;-0.006505272329987189794398005915354588069021701812744140625;0.218845268881910914871014028904028236865997314453125]
      mask Display: e = 0.06;c1 = [120 150 230]/255;c2 = ([120 150 230]+0)/383;c3 = ([120 150 230]+128)/383;patch([0 1 1 0],[0 0 1 1],c1);patch([0 1 1 1-e 1-e 0+e],[0 0 1 1-e 0+e 0+e],c2);patch([0 0 1 1-e 0+e 0+e],[0 1 1 1-e 1-e 0+e],c3);plot([0 1 1 0 0],[0 0 1 1 0]);disp('Weights');
  "IW{1,1}(9,:)'" : Constant  Value=[0.140769506868991201020691050871391780674457550048828125;-0.052305430099324430603946467499554273672401905059814453125;0.228239894339260895872456558208796195685863494873046875;-0.2032855074629895397730905415301094762980937957763671875;-0.2353357929688953686930830144774517975747585296630859375;0.21732210000781393421931397824664600193500518798828125;-0.13560155190645739597954388955258764326572418212890625;0.53432844055857897647143772701383568346500396728515625;0.297239033826869947230164825668907724320888519287109375;-0.51013915926667341427247492902097292244434356689453125;-0.02066880568600666656653430663936887867748737335205078125;-0.2512494486436678275964595741243101656436920166015625]
      mask Display: e = 0.06;c1 = [120 150 230]/255;c2 = ([120 150 230]+0)/383;c3 = ([120 150 230]+128)/383;patch([0 1 1 0],[0 0 1 1],c1);patch([0 1 1 1-e 1-e 0+e],[0 0 1 1-e 0+e 0+e],c2);patch([0 0 1 1-e 0+e 0+e],[0 1 1 1-e 1-e 0+e],c3);plot([0 1 1 0 0],[0 0 1 1 0]);disp('Weights');
  Mux : Mux  Inputs=30
      mask Display: e = 0.06;c1 = [120 150 230]/255;c2 = ([120 150 230]+0)/383;c3 = ([120 150 230]+128)/383;patch([0 1 1 0],[0 0 1 1],c1);patch([0 1 1 1-e 1-e 0+e],[0 0 1 1-e 0+e 0+e],c2);patch([0 0 1 1-e 0+e 0+e],[0 1 1 1-e 1-e 0+e],c3);plot([0 1 1 0 0],[0 0 1 1 0]);disp('Mux');
  dotprod{1..30} (30 alike) : neural/Weight Functions/dotprod
  "iz{1,1}" : Outport
      mask Display: e = 0.06;c1 = [120 230 180]/255;c2 = ([120 230 180]+0)/(256+128);c3 = ([120 230 180]+128)/(256+128);patch([0 1 1 0],[0 0 1 1],c1);patch([0 1 1 1-e 1-e 0+e],[0 0 1 1-e 0+e 0+e],c2);patch([0 0 1 1-e 0+e 0+e],[0 1 1 1-e 1-e 0+e],c3);plot([0 1 1 0 0],[0 0 1 1 0]);
  wires:
  "IW{1,1}(1,:)'"/1 -> dotprod1/1
  "pd{1,1}"/1 -> dotprod1/2, dotprod2/2, dotprod3/2, dotprod4/2, dotprod5/2, dotprod6/2, dotprod7/2, dotprod8/2, dotprod9/2, dotprod10/2, dotprod11/2, dotprod12/2, dotprod13/2, dotprod14/2, dotprod15/2, dotprod16/2, dotprod17/2, dotprod18/2, dotprod19/2, dotprod20/2, dotprod21/2, dotprod22/2, dotprod23/2, dotprod24/2, dotprod25/2, dotprod26/2, dotprod27/2, dotprod28/2, dotprod29/2, dotprod30/2
  dotprod1/1 -> Mux/1
  "IW{1,1}(2,:)'"/1 -> dotprod2/1
  dotprod2/1 -> Mux/2
  "IW{1,1}(3,:)'"/1 -> dotprod3/1
  dotprod3/1 -> Mux/3
  "IW{1,1}(4,:)'"/1 -> dotprod4/1
  dotprod4/1 -> Mux/4
  "IW{1,1}(5,:)'"/1 -> dotprod5/1
  dotprod5/1 -> Mux/5
  "IW{1,1}(6,:)'"/1 -> dotprod6/1
  dotprod6/1 -> Mux/6
  "IW{1,1}(7,:)'"/1 -> dotprod7/1
  dotprod7/1 -> Mux/7
  "IW{1,1}(8,:)'"/1 -> dotprod8/1
  dotprod8/1 -> Mux/8
  "IW{1,1}(9,:)'"/1 -> dotprod9/1
  dotprod9/1 -> Mux/9
  "IW{1,1}(10,:)'"/1 -> dotprod10/1
  dotprod10/1 -> Mux/10
  "IW{1,1}(11,:)'"/1 -> dotprod11/1
  dotprod11/1 -> Mux/11
  "IW{1,1}(12,:)'"/1 -> dotprod12/1
  dotprod12/1 -> Mux/12
  "IW{1,1}(13,:)'"/1 -> dotprod13/1
  dotprod13/1 -> Mux/13
  "IW{1,1}(14,:)'"/1 -> dotprod14/1
  dotprod14/1 -> Mux/14
  "IW{1,1}(15,:)'"/1 -> dotprod15/1
  dotprod15/1 -> Mux/15
  "IW{1,1}(16,:)'"/1 -> dotprod16/1
  dotprod16/1 -> Mux/16
  "IW{1,1}(17,:)'"/1 -> dotprod17/1
  dotprod17/1 -> Mux/17
  "IW{1,1}(18,:)'"/1 -> dotprod18/1
  dotprod18/1 -> Mux/18
  "IW{1,1}(19,:)'"/1 -> dotprod19/1
  dotprod19/1 -> Mux/19
  "IW{1,1}(20,:)'"/1 -> dotprod20/1
  dotprod20/1 -> Mux/20
  "IW{1,1}(21,:)'"/1 -> dotprod21/1
  dotprod21/1 -> Mux/21
  "IW{1,1}(22,:)'"/1 -> dotprod22/1
  dotprod22/1 -> Mux/22
  "IW{1,1}(23,:)'"/1 -> dotprod23/1
  dotprod23/1 -> Mux/23
  "IW{1,1}(24,:)'"/1 -> dotprod24/1
  dotprod24/1 -> Mux/24
  "IW{1,1}(25,:)'"/1 -> dotprod25/1
  dotprod25/1 -> Mux/25
  "IW{1,1}(26,:)'"/1 -> dotprod26/1
  dotprod26/1 -> Mux/26
  "IW{1,1}(27,:)'"/1 -> dotprod27/1
  dotprod27/1 -> Mux/27
  "IW{1,1}(28,:)'"/1 -> dotprod28/1
  dotprod28/1 -> Mux/28
  "IW{1,1}(29,:)'"/1 -> dotprod29/1
  dotprod29/1 -> Mux/29
  "IW{1,1}(30,:)'"/1 -> dotprod30/1
  dotprod30/1 -> Mux/30
  Mux/1 -> "iz{1,1}"/1

== system quad_1_ref_NN/nn_1_const/Layer 2/Delays 1 ==
  "p{2}" : Inport  PortDimensions=30
      mask Display: e = 0.06;c1 = [120 230 180]/255;c2 = ([120 230 180]+0)/(256+128);c3 = ([120 230 180]+128)/(256+128);patch([0 1 1 0],[0 0 1 1],c1);patch([0 1 1 1-e 1-e 0+e],[0 0 1 1-e 0+e 0+e],c2);patch([0 0 1 1-e 0+e 0+e],[0 1 1 1-e 1-e 0+e],c3);plot([0 1 1 0 0],[0 0 1 1 0]);
  mux : Mux  Inputs=1
      mask Display: e = 0.06;c1 = [120 150 230]/255;c2 = ([120 150 230]+0)/383;c3 = ([120 150 230]+128)/383;patch([0 1 1 0],[0 0 1 1],c1);patch([0 1 1 1-e 1-e 0+e],[0 0 1 1-e 0+e 0+e],c2);patch([0 0 1 1-e 0+e 0+e],[0 1 1 1-e 1-e 0+e],c3);plot([0 1 1 0 0],[0 0 1 1 0]);disp('Mux')
  "pd{2,1}" : Outport
      mask Display: e = 0.06;c1 = [120 230 180]/255;c2 = ([120 230 180]+0)/(256+128);c3 = ([120 230 180]+128)/(256+128);patch([0 1 1 0],[0 0 1 1],c1);patch([0 1 1 1-e 1-e 0+e],[0 0 1 1-e 0+e 0+e],c2);patch([0 0 1 1-e 0+e 0+e],[0 1 1 1-e 1-e 0+e],c3);plot([0 1 1 0 0],[0 0 1 1 0]);
  wires:
  "p{2}"/1 -> mux/1
  mux/1 -> "pd{2,1}"/1
